simulink model "theorem_1"  (R2018a)
settings: Solver=VariableStepAuto  StartTime=0.0  StopTime=10.0  RelTol=1e-3
undefined symbols (not defined in the file): A, B, N, P, Q, Vs, x0, xe
settings Model: Creator=julio  LastModifiedBy=julio

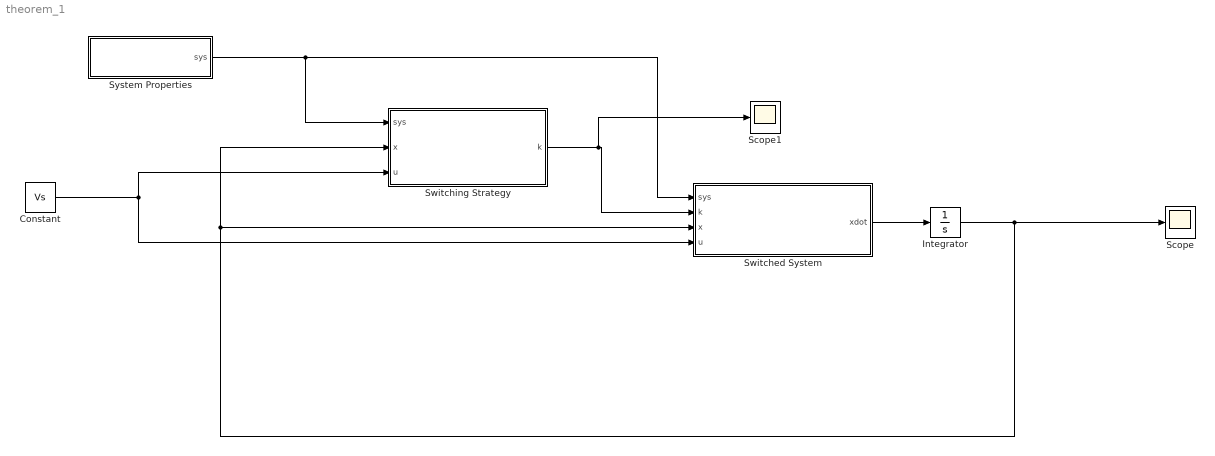
== system theorem_1 ==
  Constant : Constant  Value=Vs
  Integrator : Integrator  InitialCondition=x0
  Scope : Scope
  Scope1 : Scope
  Switched System : MATLAB Function  TreatAsAtomicUnit=on
  Switching Strategy : MATLAB Function  TreatAsAtomicUnit=on
  System Properties : Subsystem
  wires:
  Switched System/1(xdot) -> Integrator/1
  Integrator/1 -> Scope/1, Switched System/3(x), Switching Strategy/2(x)
  Constant/1 -> Switched System/4(u), Switching Strategy/3(u)
  System Properties/1(sys) -> Switched System/1(sys), Switching Strategy/1(sys)
  Switching Strategy/1(k) -> Scope1/1, Switched System/2(k)

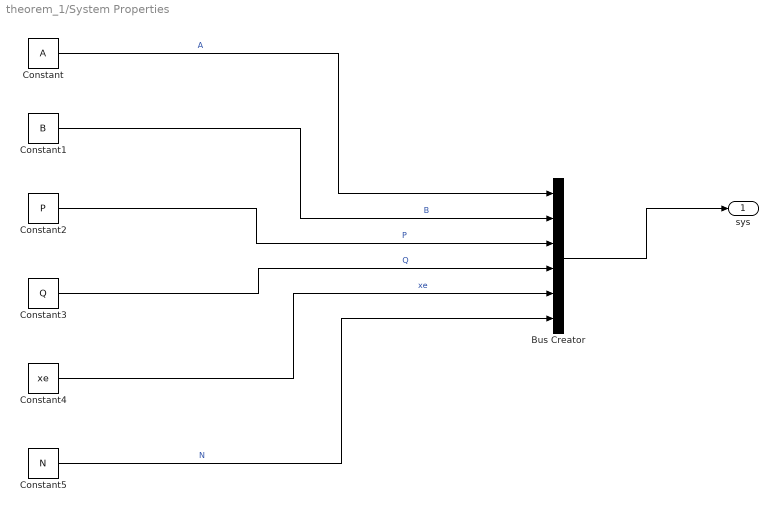
== system theorem_1/System Properties ==
  Bus Creator : BusCreator  Inputs=6  OutDataTypeStr=Bus: SystemDataBus
  Constant : Constant  Value=A
  Constant1 : Constant  Value=B
  Constant2 : Constant  Value=P
  Constant3 : Constant  Value=Q
  Constant4 : Constant  Value=xe
  Constant5 : Constant  Value=N
  sys : Outport
  wires:
  Bus Creator/1 -> sys/1
  Constant2/1 -> Bus Creator/3  "P"
  Constant1/1 -> Bus Creator/2  "B"
  Constant/1 -> Bus Creator/1  "A"
  Constant3/1 -> Bus Creator/4  "Q"
  Constant4/1 -> Bus Creator/5  "xe"
  Constant5/1 -> Bus Creator/6  "N"

== matlab function theorem_1/Switched System ==
  data: sys input; k input; x input; u input; xdot output
function xdot = switched_system(sys, k, x, u)
    xdot = sys.A(:,:,k)*x + sys.B(:,:,k)*u;
end

== matlab function theorem_1/Switching Strategy ==
  data: sys input; x input; u input; k output
function k = switching_strategy(sys, x, u)
    qsi = x - sys.xe;
    sig = zeros(sys.N,1);
    for i=1:sys.N
        sig(i) = qsi'*(sys.Q(:,:,i)*qsi + 2*sys.P*(sys.A(:,:,i)*x + sys.B(:,:,i)*u));
    end
    [~, k] = min(sig);
end
